simulink model "Kp_Effect"  (R2024b)
settings: Solver=FixedStepAuto  StartTime=0.0  StopTime=70  FixedStep=0.00001  RelTol=1e-3
settings Model: Creator=abdal  LastModifiedBy=abdal

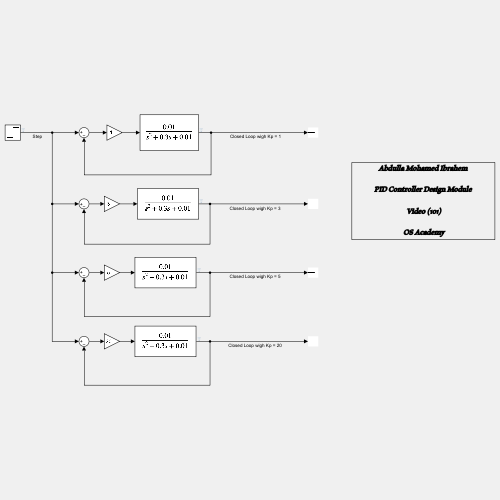
[thumbnail: Simulink's stored preview of the top-level diagram]
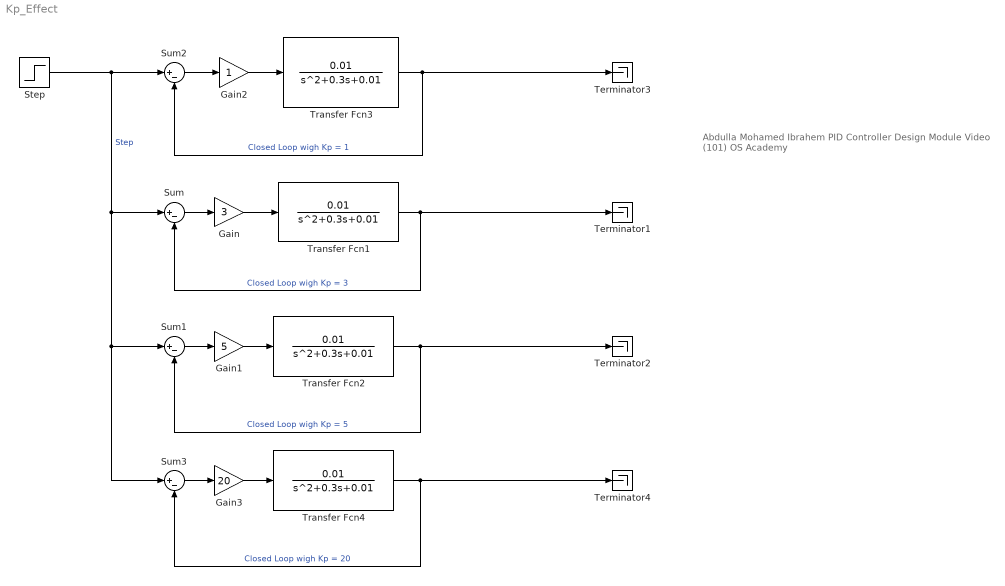
== system Kp_Effect ==
  note: Abdulla Mohamed Ibrahem
      | PID Controller Design Module
      | Video (101)
      | OS Academy
  Gain : Gain  Gain=3
  Gain1 : Gain  Gain=5
  Gain2 : Gain
  Gain3 : Gain  Gain=20
  Step : Step  SampleTime=0
  Sum{,1..3} (4 alike) : Sum  Inputs=|+-
  Terminator{1..4} (4 alike) : Terminator
  Transfer Fcn{1..4} (4 alike) : TransferFcn  Numerator=0.01  Denominator=[1 0.3 0.01]
  wires:
  Sum/1 -> Gain/1
  Transfer Fcn1/1 -> Terminator1/1, Sum/2  "Closed Loop wigh Kp = 3"
  Gain/1 -> Transfer Fcn1/1
  Gain1/1 -> Transfer Fcn2/1
  Transfer Fcn2/1 -> Terminator2/1, Sum1/2  "Closed Loop wigh Kp = 5"
  Sum1/1 -> Gain1/1
  Gain2/1 -> Transfer Fcn3/1
  Transfer Fcn3/1 -> Terminator3/1, Sum2/2  "Closed Loop wigh Kp = 1"
  Sum2/1 -> Gain2/1
  Step/1 -> Sum2/1, Sum3/1, Sum1/1, Sum/1  "Step"
  Sum3/1 -> Gain3/1
  Transfer Fcn4/1 -> Sum3/2, Terminator4/1  "Closed Loop wigh Kp = 20"
  Gain3/1 -> Transfer Fcn4/1
